simulink model "cstrpid"  (R2020a)
settings: Solver=VariableStepAuto  StartTime=0.0  StopTime=7200  RelTol=1e-3
values from neighbouring files (symbols this model uses):
  Ca0f = entrada(6)    [icstrex.m]
  Ca0i = entrada(5)    [icstrex.m]
  f0f = entrada(3)    [icstrex.m]
  f0i = entrada(2)    [icstrex.m]
  hspf = control(16)    [icstrex.m]
  hspi = control(15)    [icstrex.m]
  kd1 = control(5)    [icstrex.m]
  kd2 = control(9)    [icstrex.m]
  ki1 = control(6)    [icstrex.m]
  ki2 = control(10)    [icstrex.m]
  kp1 = control(4)    [icstrex.m]
  kp2 = control(8)    [icstrex.m]
  N1 = control(7)    [icstrex.m]
  T0 = entrada(7)    [icstrex.m]
  t_ca0 = entrada(4)    [icstrex.m]
  t_sf0 = entrada(1)    [icstrex.m]
  Tj0 = entrada(8)    [icstrex.m]
  tsp_h = control(17)    [icstrex.m]
  tsp_t = control(14)    [icstrex.m]
  Tspf = control(13)    [icstrex.m]
  Tspi = control(12)    [icstrex.m]
undefined symbols (not defined in the file or in its folder): inicial
libraries: simulink x2
settings Model: Creator=sho  LastModifiedBy=sho
settings DataIOCC: SaveFormat=Structure

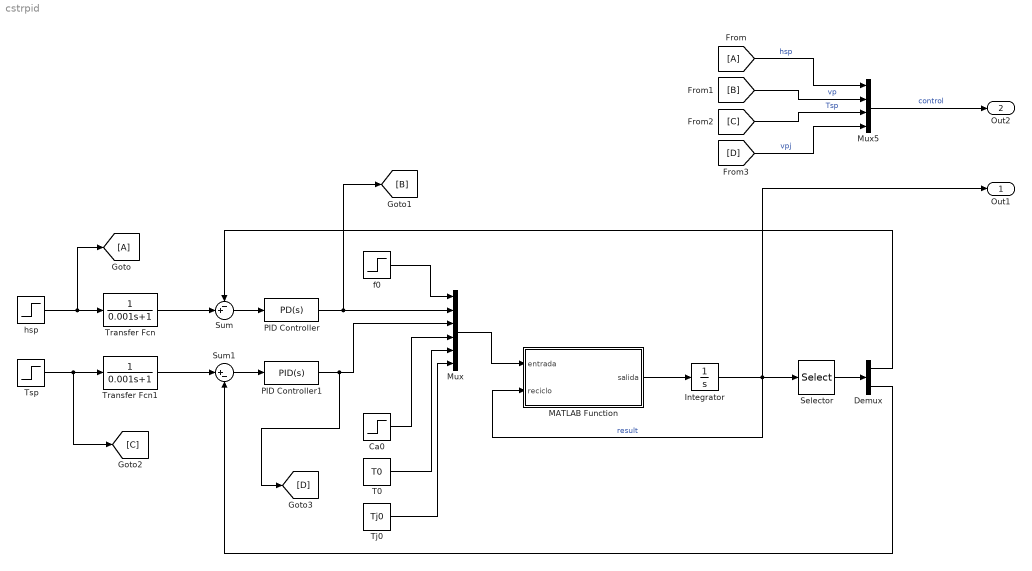
== system cstrpid ==
  Ca0 : Step  Time=t_ca0  Before=Ca0i  After=Ca0f  SampleTime=0
  Demux : Demux  Outputs=2
  Integrator : Integrator  InitialCondition=inicial
  MATLAB Function : MATLAB Function  TreatAsAtomicUnit=on
  Mux : Mux  Inputs=6
  Mux5 : Mux
  PID Controller : simulink/Continuous/PID Controller  Controller=PD  Form=Parallel  TimeDomain=Continuous-time  UseExternalTs=off  SampleTime=-1  IntegratorMethod=Forward Euler  FilterMethod=Forward Euler  ControllerParametersSource=internal  P=kp2  I=ki2  D=kd2  UseFilter=on  N=100  TunerSelectOption=Transfer Function Based (PID Tuner App)  InitialConditionSource=internal  InitialConditionForIntegrator=0  InitialConditionForFilter=0  DifferentiatorICPrevScaledInput=0  ExternalReset=none  TrackingMode=off  Kt=1  LimitOutput=on  UpperSaturationLimit=100  LowerSaturationLimit=0  LinearizeAsGain=on  AntiWindupMode=none  Kb=1  POutMin=[]  POutMax=[]  IOutMin=[]  IOutMax=[]  DOutMin=[]  DOutMax=[]  NOutMin=[]  NOutMax=[]  SumOutMin=[]  SumOutMax=[]  SaturationOutMin=[]  SaturationOutMax=[]  PParamMin=[]  PParamMax=[]  IParamMin=[]  IParamMax=[]  DParamMin=[]  DParamMax=[]  NParamMin=[]  NParamMax=[]  KbParamMin=[]  KbParamMax=[]  KtParamMin=[]  KtParamMax=[]  KbOutMin=[]  KbOutMax=[]  KtOutMin=[]  KtOutMax=[]  IntegratorOutMin=[]  IntegratorOutMax=[]  FilterOutMin=[]  FilterOutMax=[]  SumI1OutMin=[]  SumI1OutMax=[]  SumI2OutMin=[]  SumI2OutMax=[]  SumI3OutMin=[]  SumI3OutMax=[]  SumI4OutMin=[]  SumI4OutMax=[]  SumDOutMin=[]  SumDOutMax=[]  DifferentiatorOutMin=[]  DifferentiatorOutMax=[]  FilterDiffOutCoefMin=[]  FilterDiffOutCoefMax=[]  ReciprocalOutMin=[]  ReciprocalOutMax=[]  SumDenOutMin=[]  SumDenOutMax=[]  SumNumOutMin=[]  SumNumOutMax=[]  DivideOutMin=[]  DivideOutMax=[]  UdiffTsProdOutMin=[]  UdiffTsProdOutMax=[]  NTsProdOutMin=[]  NTsProdOutMax=[]  UintegralTsProdOutMin=[]  UintegralTsProdOutMax=[]  UngainTsProdOutMin=[]  UngainTsProdOutMax=[]  IntegratorContinuousStateAttributes=''  IntegratorStateMustResolveToSignalObject=off  IntegratorRTWStateStorageClass=Auto  FilterContinuousStateAttributes=''  FilterStateMustResolveToSignalObject=off  FilterRTWStateStorageClass=Auto  ParallelPVariant=InternalParameters  IdealPVariant=Disabled  IVariant=Disabled  DVariant=InternalParameters  IntegratorVariant=Disabled  SatVariant=Enabled  AWVariant=Disabled  PCopyVariant=Disabled  TRVariant=Disabled  FdbkBlocksVariant=Forward  IdealPFdbkVariant=Disabled  SatFdbkVariant=Disabled  DerivativeFilterVariant=ContFilter  NVariant=InternalParameters  NCopyVariant=Disabled  FilterICVariant=InternalICsFilter  IntegratorICVariant=Disabled  ExternalResetVariant=Disabled  TRSumVariant=Passthrough  SumFdbkVariant=Disabled  SumVariant=Sum_PD  TsampFilterVariant=InternalTs  TsampNgainVariant=Passthrough  TsampIntegralVariant=Disabled_SignalSpec
  PID Controller1 : simulink/Continuous/PID Controller  Controller=PID  Form=Parallel  TimeDomain=Continuous-time  UseExternalTs=off  SampleTime=-1  IntegratorMethod=Forward Euler  FilterMethod=Forward Euler  ControllerParametersSource=internal  P=kp1  I=ki1  D=kd1  UseFilter=on  N=N1  TunerSelectOption=Frequency Response Based  InitialConditionSource=internal  InitialConditionForIntegrator=0  InitialConditionForFilter=0  DifferentiatorICPrevScaledInput=0  ExternalReset=none  TrackingMode=off  Kt=1  LimitOutput=on  UpperSaturationLimit=1  LowerSaturationLimit=0  LinearizeAsGain=on  AntiWindupMode=none  Kb=1  POutMin=[]  POutMax=[]  IOutMin=[]  IOutMax=[]  DOutMin=[]  DOutMax=[]  NOutMin=[]  NOutMax=[]  SumOutMin=[]  SumOutMax=[]  SaturationOutMin=[]  SaturationOutMax=[]  PParamMin=[]  PParamMax=[]  IParamMin=[]  IParamMax=[]  DParamMin=[]  DParamMax=[]  NParamMin=[]  NParamMax=[]  KbParamMin=[]  KbParamMax=[]  KtParamMin=[]  KtParamMax=[]  KbOutMin=[]  KbOutMax=[]  KtOutMin=[]  KtOutMax=[]  IntegratorOutMin=[]  IntegratorOutMax=[]  FilterOutMin=[]  FilterOutMax=[]  SumI1OutMin=[]  SumI1OutMax=[]  SumI2OutMin=[]  SumI2OutMax=[]  SumI3OutMin=[]  SumI3OutMax=[]  SumI4OutMin=[]  SumI4OutMax=[]  SumDOutMin=[]  SumDOutMax=[]  DifferentiatorOutMin=[]  DifferentiatorOutMax=[]  FilterDiffOutCoefMin=[]  FilterDiffOutCoefMax=[]  ReciprocalOutMin=[]  ReciprocalOutMax=[]  SumDenOutMin=[]  SumDenOutMax=[]  SumNumOutMin=[]  SumNumOutMax=[]  DivideOutMin=[]  DivideOutMax=[]  UdiffTsProdOutMin=[]  UdiffTsProdOutMax=[]  NTsProdOutMin=[]  NTsProdOutMax=[]  UintegralTsProdOutMin=[]  UintegralTsProdOutMax=[]  UngainTsProdOutMin=[]  UngainTsProdOutMax=[]  IntegratorContinuousStateAttributes=''  IntegratorStateMustResolveToSignalObject=off  IntegratorRTWStateStorageClass=Auto  FilterContinuousStateAttributes=''  FilterStateMustResolveToSignalObject=off  FilterRTWStateStorageClass=Auto  ParallelPVariant=InternalParameters  IdealPVariant=Disabled  IVariant=InternalParameters  DVariant=InternalParameters  IntegratorVariant=Continuous  SatVariant=Enabled  AWVariant=Passthrough  PCopyVariant=Disabled  TRVariant=Disabled  FdbkBlocksVariant=Forward  IdealPFdbkVariant=Disabled  SatFdbkVariant=Disabled  DerivativeFilterVariant=ContFilter  NVariant=InternalParameters  NCopyVariant=Disabled  FilterICVariant=InternalICsFilter  IntegratorICVariant=InternalICs  ExternalResetVariant=Disabled  TRSumVariant=Passthrough  SumFdbkVariant=Disabled  SumVariant=Sum_PID  TsampFilterVariant=InternalTs  TsampNgainVariant=Passthrough  TsampIntegralVariant=Passthrough
  Selector : Selector  InputPortWidth=5  IndexOptions=Index vector (dialog)  Indices=[1 4]  OutputSizes=1
  Sum : Sum  Inputs=-+|
  Sum1 : Sum  Inputs=|+-
  T0 : Constant  Value=T0
  Tj0 : Constant  Value=Tj0
  Transfer Fcn : TransferFcn  Denominator=[0.001 1]
  Transfer Fcn1 : TransferFcn  Denominator=[0.001 1]
  Tsp : Step  Time=tsp_t  Before=Tspi  After=Tspf  SampleTime=0
  f0 : Step  Time=t_sf0  Before=f0i  After=f0f  SampleTime=0
  hsp : Step  Time=tsp_h  Before=hspi  After=hspf  SampleTime=0
  Out1 : Outport
  Out2 : Outport  Port=2
  wires:
  MATLAB Function/1(salida) -> Integrator/1
  Mux/1 -> MATLAB Function/1(entrada)
  Integrator/1 -> Out1/1, Selector/1, MATLAB Function/2(reciclo)  "result"
  f0/1 -> Mux/1
  Ca0/1 -> Mux/4
  T0/1 -> Mux/5
  Tj0/1 -> Mux/6
  hsp/1 -> [A], Transfer Fcn/1
  Tsp/1 -> [C], Transfer Fcn1/1
  PID Controller/1 -> [B], Mux/2
  PID Controller1/1 -> [D], Mux/3
  Transfer Fcn/1 -> Sum/2
  Transfer Fcn1/1 -> Sum1/1
  Sum1/1 -> PID Controller1/1
  Sum/1 -> PID Controller/1
  Mux5/1 -> Out2/1  "control"
  Selector/1 -> Demux/1
  Demux/1 -> Sum/1
  Demux/2 -> Sum1/2
  [A] -> Mux5/1  "hsp"
  [B] -> Mux5/2  "vp"
  [C] -> Mux5/3  "Tsp"
  [D] -> Mux5/4  "vpj"

== matlab function cstrpid/MATLAB Function ==
  data: entrada input size=6; salida output size=5; reciclo input size=5; constantes parameter
function salida = cstriex(entrada, reciclo, constantes)

% Entradas
f0 = entrada(1,1);
vp = entrada(2,1);
vpj = entrada(3,1);
Ca0 = entrada(4,1);
T0 = entrada(5,1);
Tj0 = entrada(6,1);

% Reciclo
h = reciclo(1);
Ca = reciclo(2);
Cb = reciclo(3);
T = reciclo(4);
Tj = reciclo(5);

% Constant
k0 = constantes(1);
k1 = constantes(2);
k2 = constantes(3);
k3 = constantes(4);
k4 = constantes(5);
k5 = constantes(6);
k6 = constantes(7);
k7 = constantes(8);
k8 = constantes(9);

% Flujo de salida del reactor
f = k7*sqrt(h)*vp;

% Flujo de entrada de agua - chaqueta
fj = k8*vpj;

% La constante cinética
kt = k0*exp(-k6/T);

% Balance de masa general
dh = k1*(f0 - f); 

% Balance del componente A
dCa = (((k1*f0)/h)*(Ca0-Ca))-(kt*Ca);

% Balance del componente B
dCb = (kt*Ca)-(k1*f0*Cb)/h;

% Balance de energía en el reactor
dT = ((k1*f0)/h)*(T0-T) - ((k2/h)*(T-Tj)) - (k3*kt*Ca);

% Balance de energía en la chaqueta
dTj = (k4*fj*(Tj0-Tj)) +(k5*(T-Tj));

salida = [dh; dCa; dCb; dT; dTj];
